simulink model "myfirstblinker"  (R2018b)
settings: Solver=VariableStepAuto  StartTime=0.0  StopTime=Inf  RelTol=1e-3
settings Model: Creator=Sjoerd  LastModifiedBy=Sjoerd

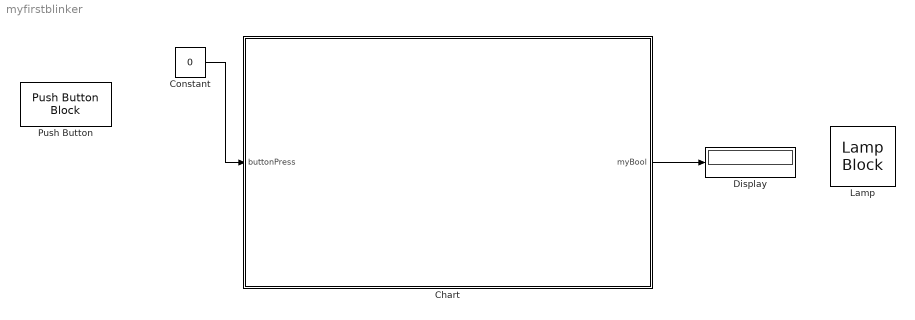
== system myfirstblinker ==
  Chart : Stateflow chart  TreatAsAtomicUnit=on
  Constant : Constant  Value=0
  Display : Display
  Lamp : LampBlock  WebBlockId=4
  Push Button : PushButtonBlock  WebBlockId=2
  wires:
  Constant/1 -> Chart/1(buttonPress)
  Chart/1(myBool) -> Display/1

== stateflow chart myfirstblinker/Chart ==
  state NotPressed
  state Pressed
  (default) -> NotPressed : {myBool = 0}
  NotPressed -> Pressed : [buttonPress == 1]{myBool = 1}
  Pressed -> NotPressed : [buttonPress == 0]{myBool = 0}
  data: buttonPress input; myBool output
